simulink model "frictionmodel"  (R2018b)
settings: configuration reference "Physics" (kept outside this file)
model workspace (MAT data in the model file):
  veh_param = Simulink.Parameter
  veh_param.Value.cLiftF = 0
  veh_param.Value.cLiftR = 0
  veh_param.Value.CoGx_m = 0
  veh_param.Value.CoGy_m = 0
  veh_param.Value.CoGz_m = 0
  veh_param.Value.cDrag = 0
  veh_param.Value.Aref_m2 = 0
  veh_param.Value.Gearratio = 0
  veh_param.Value.Wheelbase_m = 0
  veh_param.Value.PacLatF = [0 0 0 0 0]
  veh_param.Value.PacLongF = [0 0 0 0 0]
  veh_param.Value.PacLatR = [0 0 0 0 0]
  veh_param.Value.PacLongR = [0 0 0 0 0]
  veh_param.Value.cRollFriction_Npmps = 0
  veh_param.Value.MaxRollFriction_N = 0
  veh_param.Value.T_YawRate_s = 0
  veh_param.Value.T_LatVel_s = 0
  veh_param.Value.TrackWidthF_m = 0
  veh_param.Value.TrackWidthR_m = 0
  veh_param.Value.TireRadiusF_m = 0
  veh_param.Value.TireRadiusR_m = 0
  veh_param.Value.VehicleInertia_kgm2 = 0
  veh_param.Value.WheelInertiaF_kgm2 = 0
  veh_param.Value.WheelInertiaR_kgm2 = 0
  veh_param.Value.VehicleMass_kg = 0
  veh_param.Value.switchModelBlend_mps = 0
  veh_param.Value.PTLimitLowVel_N = 0
  veh_param.Value.switchModelVel_mps = 0
  veh_param.Value.T_Tire_s = 0
  veh_param.DataType = 'struct'
  veh_param.Dimensions = [1 1]
  x0_positionstates = Simulink.Parameter
  x0_positionstates.Value = [0 0 0]
  x0_positionstates.DataType = 'auto'
  x0_positionstates.Dimensions = [1 3]
undefined symbols (not defined in the file): Grid_map_1, Grid_map_2, Grid_map_3, Grid_map_4, Gridmap_Ident
settings Model: DataDictionary=frictionmodel.sldd  OrderedModelArguments=off  Creator=wischnewski  LastModifiedBy=staer

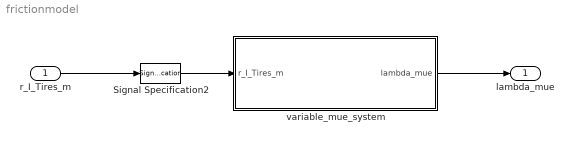
== system frictionmodel ==
  r_I_Tires_m : Inport
  Signal Specification2 : SignalSpecification  Dimensions=[3,4]
  variable_mue_system : Subsystem  VariantControl=activate_VariableFriction==1
  lambda_mue : Outport
  wires:
  variable_mue_system/1(lambda_mue) -> lambda_mue/1
  r_I_Tires_m/1 -> Signal Specification2/1
  Signal Specification2/1 -> variable_mue_system/1(r_I_Tires_m)

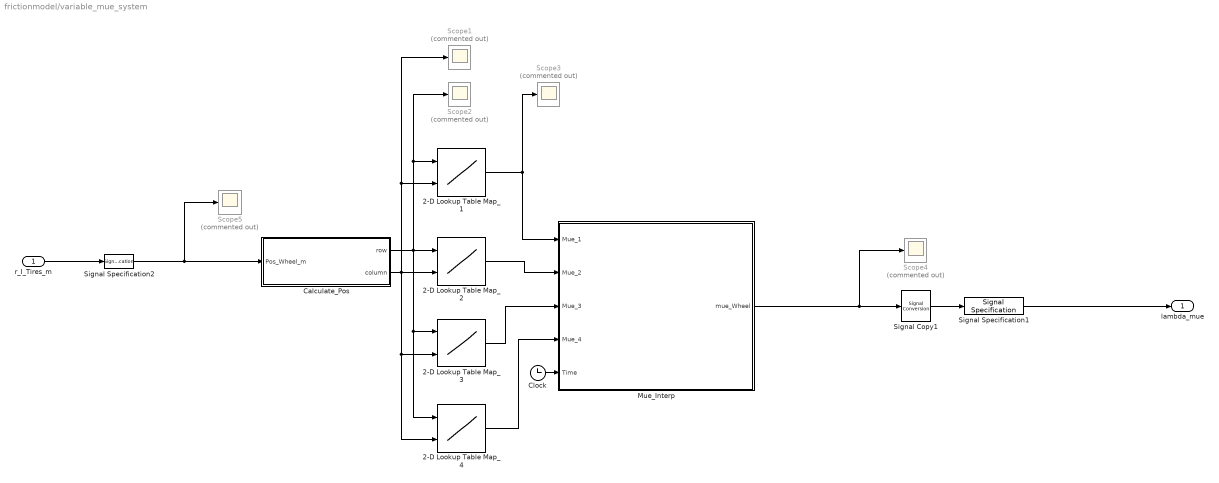
== system frictionmodel/variable_mue_system ==
  r_I_Tires_m : Inport
  2-D Lookup Table Map_1 : Lookup_n-D  BreakpointsForDimension1=[1:Gridmap_Ident(3,1)]  BreakpointsForDimension2=[1:Gridmap_Ident(3,2)]  Table=Grid_map_1  InternalRulePriority=Speed  RndMeth=Simplest  InputSameDT=on
  2-D Lookup Table Map_2 : Lookup_n-D  BreakpointsForDimension1=[1:Gridmap_Ident(3,1)]  BreakpointsForDimension2=[1:Gridmap_Ident(3,2)]  Table=Grid_map_2  InternalRulePriority=Speed  RndMeth=Simplest  InputSameDT=on
  2-D Lookup Table Map_3 : Lookup_n-D  BreakpointsForDimension1=[1:Gridmap_Ident(3,1)]  BreakpointsForDimension2=[1:Gridmap_Ident(3,2)]  Table=Grid_map_3  InternalRulePriority=Speed  RndMeth=Simplest  InputSameDT=on
  2-D Lookup Table Map_4 : Lookup_n-D  BreakpointsForDimension1=[1:Gridmap_Ident(3,1)]  BreakpointsForDimension2=[1:Gridmap_Ident(3,2)]  Table=Grid_map_4  InternalRulePriority=Speed  RndMeth=Simplest  InputSameDT=on
  Calculate_Pos : MATLAB Function  TreatAsAtomicUnit=on
  Clock : Clock
  Mue_Interp : MATLAB Function  TreatAsAtomicUnit=on
  Scope{1..5} (5 alike) : Scope  Commented=on
  Signal Copy1 : SignalConversion  OverrideOpt=off
  Signal Specification1 : SignalSpecification  Dimensions=[1,4]
  Signal Specification2 : SignalSpecification  Dimensions=[3,4]
  lambda_mue : Outport
  wires:
  Clock/1 -> Mue_Interp/5(Time)
  r_I_Tires_m/1 -> Signal Specification2/1
  Signal Copy1/1 -> Signal Specification1/1
  Signal Specification2/1 -> Calculate_Pos/1(Pos_Wheel_m), Scope5/1
  Calculate_Pos/2(column) -> Scope1/1, 2-D Lookup Table Map_1/2, 2-D Lookup Table Map_4/2, 2-D Lookup Table Map_3/2, 2-D Lookup Table Map_2/2
  2-D Lookup Table Map_1/1 -> Mue_Interp/1(Mue_1), Scope3/1
  2-D Lookup Table Map_2/1 -> Mue_Interp/2(Mue_2)
  2-D Lookup Table Map_3/1 -> Mue_Interp/3(Mue_3)
  2-D Lookup Table Map_4/1 -> Mue_Interp/4(Mue_4)
  Mue_Interp/1(mue_Wheel) -> Scope4/1, Signal Copy1/1
  Calculate_Pos/1(row) -> 2-D Lookup Table Map_2/1, Scope2/1, 2-D Lookup Table Map_1/1, 2-D Lookup Table Map_4/1, 2-D Lookup Table Map_3/1
  Signal Specification1/1 -> lambda_mue/1

== matlab function frictionmodel/variable_mue_system/Calculate_Pos ==
  data: Pos_Wheel_m input; row output; column output; Gridmap_Ident parameter
function [row, column] = fcn(Pos_Wheel_m, Gridmap_Ident)
[row, column] = Calculate_Pos(Pos_Wheel_m, Gridmap_Ident);

== matlab function frictionmodel/variable_mue_system/Mue_Interp ==
  data: Mue_1 input; mue_Wheel output; Mue_2 input; Mue_3 input; Mue_4 input; InterpTime parameter; Time input
function mue_Wheel = fcn(Mue_1, Mue_2, Mue_3, Mue_4, InterpTime, Time)
[mue_Wheel] = Mue_Interp(Mue_1, Mue_2, Mue_3, Mue_4, InterpTime, Time);
